simulink model "test"  (R2015a)
settings: Solver=FixedStepDiscrete  StartTime=0.0  StopTime=100  FixedStep=0.01  RelTol=1e-3
libraries: arduinolib x3, simulink x3
settings Model: ExtModeTrigDuration=2  Creator=pela  LastModifiedBy=pela
settings OptimizationCC: OptimizeModelRefInitCode=on  LifeSpan=1
settings DebuggingCC: UnderspecifiedInitializationDetection=Classic  MergeDetectMultiDrivingBlocksExec=none
settings HardwareCC: ProdBitPerInt=16  ProdBitPerPointer=8  ProdIntDivRoundTo=Zero  ProdEndianess=LittleEndian  ProdWordSize=8  ProdHWDeviceType=Atmel->AVR
settings RTWCC: SystemTargetFile=realtime.tlc  GenerateMakefile=off  TemplateMakefile=realtime.tmf  Description=Run on Target Hardware  RTWVerbose=off
settings ERTTargetCC: CombineOutputUpdateFcns=off  ExtModeTransport=3  ExtModeMexFile=ext_serial_win32_comm_rtt  ExtModeMexArgs=0 1 9600  ERTSrcFileBannerTemplate=realtime_code_template.cgt  ERTHdrFileBannerTemplate=realtime_code_template.cgt  ERTDataSrcFileTemplate=realtime_code_template.cgt  ERTDataHdrFileTemplate=realtime_code_template.cgt  ERTCustomFileTemplate=realtime_file_process.tlc

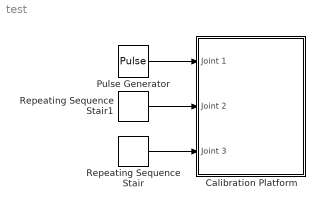
== system test ==
  Calibration Platform : Subsystem
  Pulse Generator : DiscretePulseGenerator  PulseType=Time based  Amplitude=10  Period=7*7  PulseWidth=.5/(7*7)*100
  Repeating Sequence Stair : simulink/Sources/Repeating Sequence Stair  OutValues=[90 60 30 0 -30 -60 -90]  tsamp=1  OutMin=[]  OutMax=[]  OutDataTypeStr=double  OutputDataTypeScalingMode=double  OutDataType=fixdt(0,8)  ConRadixGroup=Best Precision: Vector-wise  OutScaling=2^-12
  Repeating Sequence Stair1 : simulink/Sources/Repeating Sequence Stair  OutValues=[0 30 60 90 120 150 176]  tsamp=7  OutMin=[]  OutMax=[]  OutDataTypeStr=double  OutputDataTypeScalingMode=double  OutDataType=fixdt(0,8)  ConRadixGroup=Best Precision: Vector-wise  OutScaling=2^-12
  wires:
  Pulse Generator/1 -> Calibration Platform/1(Joint 1)
  Repeating Sequence Stair1/1 -> Calibration Platform/2(Joint 2)
  Repeating Sequence Stair/1 -> Calibration Platform/3(Joint 3)

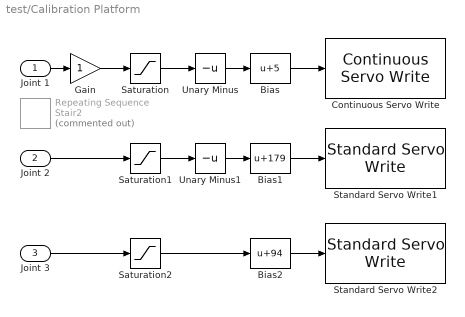
== system test/Calibration Platform ==
  Joint 1 : Inport
  Joint 2 : Inport  Port=2
  Joint 3 : Inport  Port=3
  Bias : Bias  Bias=5
  Bias1 : Bias  Bias=179
  Bias2 : Bias  Bias=94
  Continuous Servo Write : arduinolib/Continuous Servo Write  pinNumber=11  blockPlatform=arduino
  Gain : Gain
  Repeating Sequence Stair2 : simulink/Sources/Repeating Sequence Stair  Commented=on  OutValues=[0 -18 0 24 0]  tsamp=3  OutMin=[]  OutMax=[]  OutDataTypeStr=double  OutputDataTypeScalingMode=double  OutDataType=fixdt(0,8)  ConRadixGroup=Best Precision: Vector-wise  OutScaling=2^-12
  Saturation : Saturate  UpperLimit=90  LowerLimit=-90
  Saturation1 : Saturate  UpperLimit=180  LowerLimit=0
  Saturation2 : Saturate  UpperLimit=90  LowerLimit=-90
  Standard Servo Write1 : arduinolib/Standard Servo Write  pinNumber=10  blockPlatform=arduino
  Standard Servo Write2 : arduinolib/Standard Servo Write  pinNumber=9  blockPlatform=arduino
  Unary Minus : UnaryMinus
  Unary Minus1 : UnaryMinus
  wires:
  Joint 3/1 -> Saturation2/1
  Joint 1/1 -> Gain/1
  Bias/1 -> Continuous Servo Write/1
  Saturation/1 -> Unary Minus/1
  Gain/1 -> Saturation/1
  Bias1/1 -> Standard Servo Write1/1
  Saturation2/1 -> Bias2/1
  Bias2/1 -> Standard Servo Write2/1
  Unary Minus/1 -> Bias/1
  Unary Minus1/1 -> Bias1/1
  Joint 2/1 -> Saturation1/1
  Saturation1/1 -> Unary Minus1/1
